simulink model "unicycle"  (R2025b)
settings: Solver=VariableStepAuto  StartTime=0.0  StopTime=10.0  RelTol=1e-3
settings Model: Creator=Cris  LastModifiedBy=Cris
settings DebuggingCC: SignalInfNanChecking=error

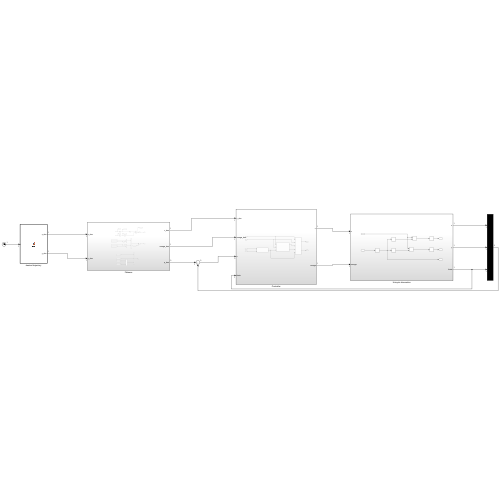
[thumbnail: Simulink's stored preview of the top-level diagram]
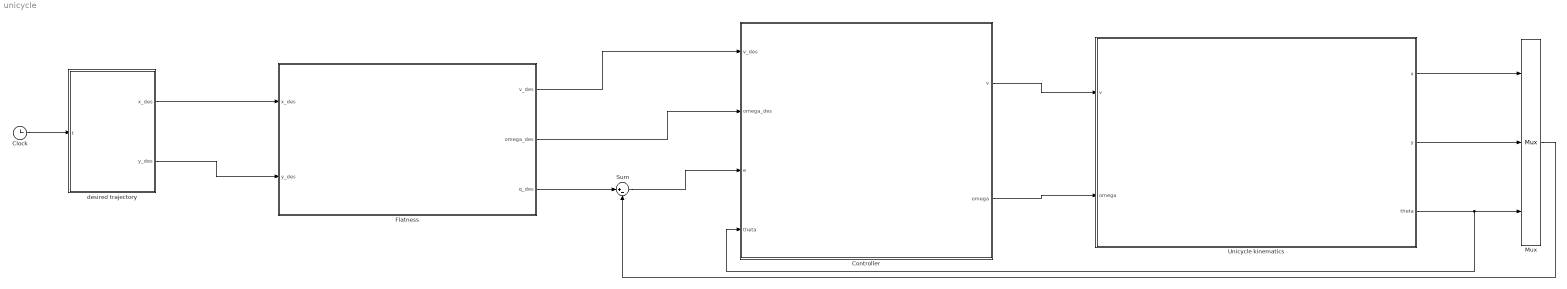
== system unicycle ==
  Clock : Clock
  Controller : Subsystem
  Flatness : Subsystem
  Mux : Mux  Inputs=3
  Sum : Sum  Inputs=|+-
  Unicycle kinematics : Subsystem
  desired trajectory : MATLAB Function  TreatAsAtomicUnit=on
  wires:
  Flatness/1(v_des) -> Controller/1(v_des)
  Flatness/2(omega_des) -> Controller/2(omega_des)
  Flatness/3(q_des) -> Sum/1
  Sum/1 -> Controller/3(e)
  Unicycle kinematics/1(x) -> Mux/1
  Unicycle kinematics/2(y) -> Mux/2
  Unicycle kinematics/3(theta) -> Controller/4(theta), Mux/3
  Mux/1 -> Sum/2
  Controller/2(omega) -> Unicycle kinematics/2(omega)
  Controller/1(v) -> Unicycle kinematics/1(v)
  Clock/1 -> desired trajectory/1(t)
  desired trajectory/1(x_des) -> Flatness/1(x_des)
  desired trajectory/2(y_des) -> Flatness/2(y_des)

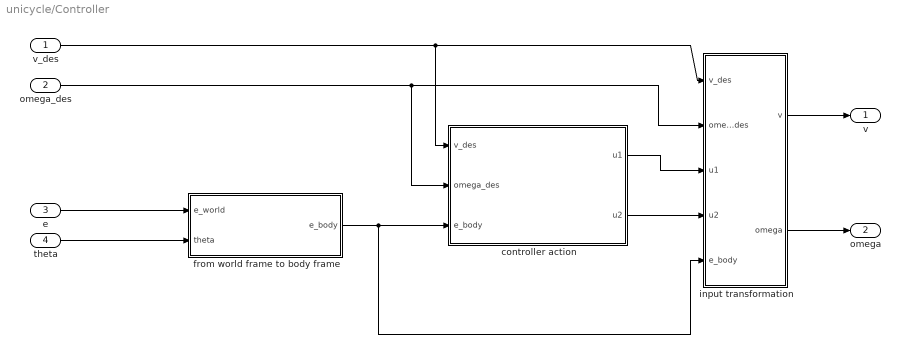
== system unicycle/Controller ==
  v_des : Inport
  omega_des : Inport  Port=2
  e : Inport  Port=3
  theta : Inport  Port=4
  controller action : MATLAB Function  TreatAsAtomicUnit=on
  from world frame to body frame : MATLAB Function  TreatAsAtomicUnit=on
  input transformation : MATLAB Function  TreatAsAtomicUnit=on
  v : Outport
  omega : Outport  Port=2
  wires:
  e/1 -> from world frame to body frame/1(e_world)
  theta/1 -> from world frame to body frame/2(theta)
  from world frame to body frame/1(e_body) -> input transformation/5(e_body), controller action/3(e_body)
  v_des/1 -> controller action/1(v_des), input transformation/1(v_des)
  controller action/2(u2) -> input transformation/4(u2)
  input transformation/2(omega) -> omega/1
  input transformation/1(v) -> v/1
  omega_des/1 -> input transformation/2(omega_des), controller action/2(omega_des)
  controller action/1(u1) -> input transformation/3(u1)

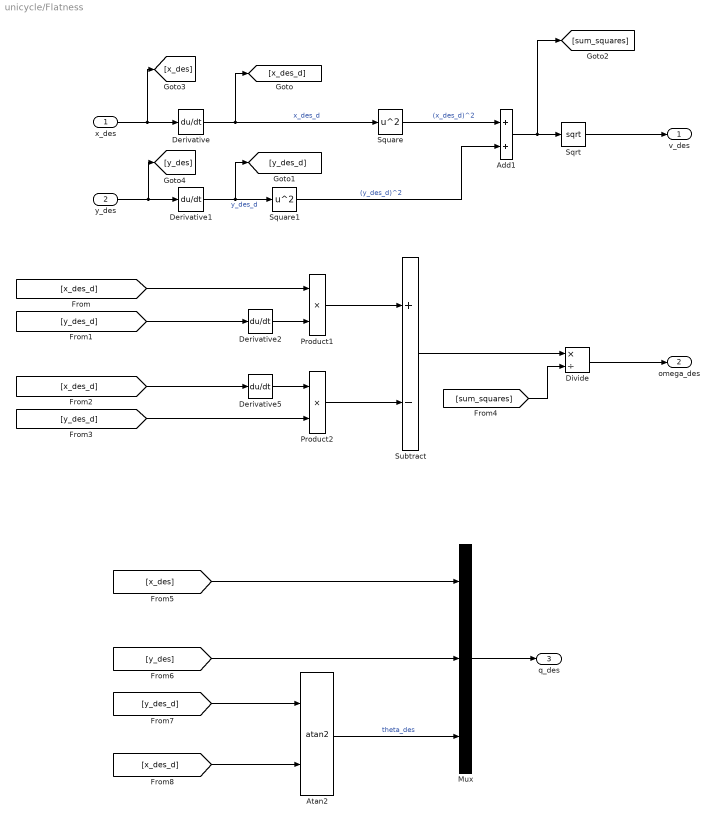
== system unicycle/Flatness ==
  x_des : Inport
  y_des : Inport  Port=2
  Add1 : Sum
  Atan2 : Trigonometry  Operator=atan2
  Derivative{,1..2,5} (4 alike) : Derivative
  Divide : Product  Inputs=*/
  Mux : Mux  Inputs=3
  Product1 : Product
  Product2 : Product
  Sqrt : Sqrt
  Square : Math  Operator=square
  Square1 : Math  Operator=square
  Subtract : Sum  Inputs=+-
  v_des : Outport
  omega_des : Outport  Port=2
  q_des : Outport  Port=3
  wires:
  x_des/1 -> [x_des], Derivative/1
  y_des/1 -> [y_des], Derivative1/1
  Derivative/1 -> [x_des_d], Square/1  "x_des_d"
  Derivative1/1 -> [y_des_d], Square1/1  "y_des_d"
  Square/1 -> Add1/1  "(x_des_d)^2"
  Square1/1 -> Add1/2  "(y_des_d)^2"
  Add1/1 -> [sum_squares], Sqrt/1
  Sqrt/1 -> v_des/1
  [x_des_d] -> Product1/1
  [y_des_d] -> Derivative2/1
  Derivative2/1 -> Product1/2
  [y_des_d] -> Product2/2
  [x_des_d] -> Derivative5/1
  Derivative5/1 -> Product2/1
  Product1/1 -> Subtract/1
  Product2/1 -> Subtract/2
  Subtract/1 -> Divide/1
  [sum_squares] -> Divide/2
  Divide/1 -> omega_des/1
  Mux/1 -> q_des/1
  [x_des] -> Mux/1
  [y_des] -> Mux/2
  Atan2/1 -> Mux/3  "theta_des"
  [x_des_d] -> Atan2/2
  [y_des_d] -> Atan2/1

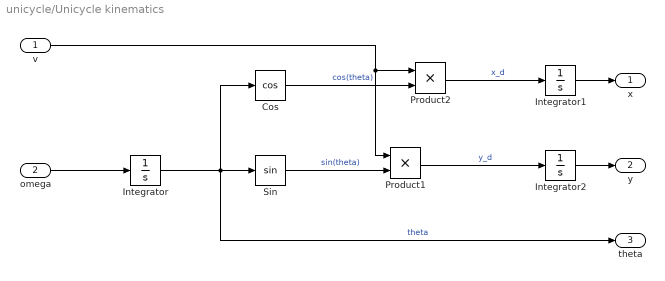
== system unicycle/Unicycle kinematics ==
  v : Inport
  omega : Inport  Port=2
  Cos : Trigonometry  Operator=cos
  Integrator : Integrator
  Integrator1 : Integrator
  Integrator2 : Integrator
  Product1 : Product
  Product2 : Product
  Sin : Trigonometry
  x : Outport
  y : Outport  Port=2
  theta : Outport  Port=3
  wires:
  omega/1 -> Integrator/1
  Integrator/1 -> theta/1, Cos/1, Sin/1  "theta"
  Cos/1 -> Product2/2  "cos(theta)"
  Sin/1 -> Product1/2  "sin(theta)"
  v/1 -> Product2/1, Product1/1
  Integrator1/1 -> x/1
  Product2/1 -> Integrator1/1  "x_d"
  Integrator2/1 -> y/1
  Product1/1 -> Integrator2/1  "y_d"

== matlab function unicycle/Controller/controller action ==
  data: v_des input; omega_des input; e_body input; u1 output; u2 output
function [u1, u2] = fcn(v_des, omega_des, e_body)

% TO DO: parametri da modfiicare
d = 1/sqrt(2);
a = 10;


% parametri controllore
k1 = 2*d*a;

if abs(v_des) < 1e-4
    if v_des >= 0
        v_des = 1e-4;
    else
        v_des = -1e-4;
    end
end

k3 = k1;
k2 = ( a^2-(omega_des)^2 ) / v_des;

u1 = [-k1, 0, 0] * e_body;
u2 = [0, -k2, -k3] * e_body;

== matlab function unicycle/Controller/from world frame to body frame ==
  data: e_world input; e_body output size=3; theta input
function e_body = fcn(e_world, theta)


% Transformation matrix
R = [cos(theta), sin(theta), 0; 
    -sin(theta), cos(theta), 0;
    0, 0, 1];

% get error in body frame
e_body = R*e_world;

== matlab function unicycle/Controller/input transformation ==
  data: v_des input; v output size=1; omega_des input; u1 input; u2 input; e_body input size=3; omega output
function [v, omega] = fcn(v_des, omega_des, u1, u2, e_body)


v = v_des * cos(e_body(3)) - u1;
omega = omega_des - u2;

== matlab function unicycle/desired trajectory ==
  data: t input; x_des output; y_des output
function [x_des, y_des] = fcn(t)

% configurable:
radius = 5;
omega_des = 1;

% desired trajectory
x_des = radius*cos(omega_des*t);
y_des = radius*sin(omega_des*t);
